simulink model "Pole_Placement_Digital_a"  (Simulink 9.0)
settings: Solver=VariableStepAuto  StartTime=0.0  StopTime=60  RelTol=1e-3
values from neighbouring files (symbols this model uses):
  C_D2 = c2d(C2_aug, T, 'tustin')    [Lab3_Pole_Placement_Integrator.m]
  K1 = 0.66538    [Lab3_Pole_Placement_Integrator.m]
  K2 = 0.062    [Lab3_Pole_Placement_Integrator.m]
  K3 = 4.78    [Lab3_Pole_Placement_Integrator.m]
  Kp = 15    [Lab3_Pole_Placement_Integrator.m]
  Kp_c2 = 2 / DC_gain    [Lab3_Pole_Placement_Integrator.m]
  p = 10.5    [Lab3_Pole_Placement_Integrator.m]
  T = 0.005    [Lab3_Pole_Placement_Integrator.m]
  tau = 0.030541    [Lab3_Pole_Placement_Integrator.m]
  z = 10    [Lab3_Pole_Placement_Integrator.m]
settings Model: Creator=joe  LastModifiedBy=joe
settings DataIOCC: SaveFormat=Dataset
settings DebuggingCC: UnderspecifiedInitializationDetection=Simplified  MergeDetectMultiDrivingBlocksExec=error  SFUnexpectedBacktrackingDiag=error  SFNoUnconditionalDefaultTransitionDiag=error
settings HardwareCC: ProdBitPerPointer=64  ProdBitPerSizeT=64  ProdBitPerPtrDiffT=64  ProdLargestAtomicFloat=Float  ProdIntDivRoundTo=Zero  ProdEndianess=LittleEndian  ProdWordSize=64  ProdHWDeviceType=Intel->x86-64 (Windows64)
settings ModelReferenceCC: PropagateSignalLabelsOutOfModel=on
settings GRTTargetCC: TargetLangStandard=C99 (ISO)
settings ConfigComp: CovMetricSettings=dwe  CovHtmlReporting=off  CovSaveCumulativeToWorkspaceVar=off  CovSaveSingleToWorkspaceVar=off  CovExternalEMLEnable=on

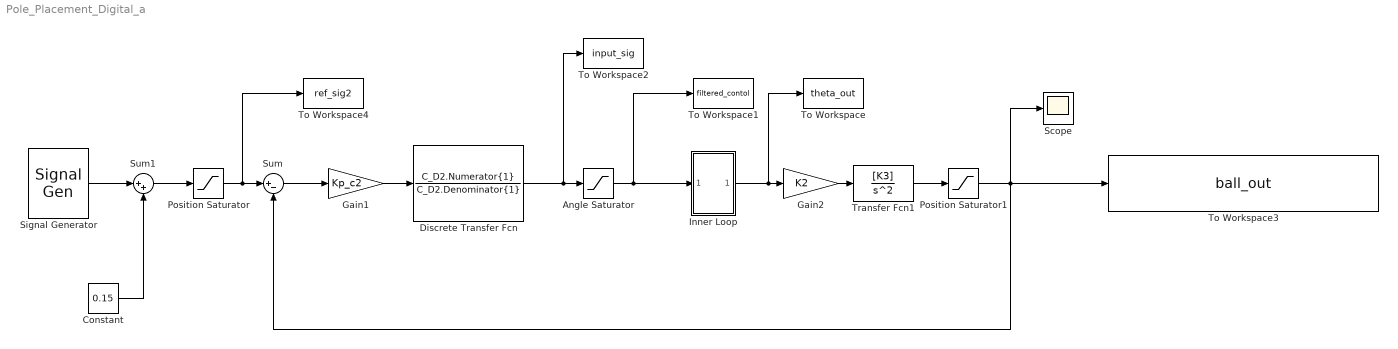
== system Pole_Placement_Digital_a ==
  Angle Saturator : Saturate  UpperLimit=0.785  LowerLimit=-0.785
  Constant : Constant  Value=0.15
  Discrete Transfer Fcn : DiscreteTransferFcn  Numerator=C_D2.Numerator{1}  Denominator=C_D2.Denominator{1}  SampleTime=T
  Gain1 : Gain  Gain=Kp_c2
  Gain2 : Gain  Gain=K2
  Inner Loop : Subsystem
  Position Saturator : Saturate  UpperLimit=0.417  LowerLimit=0
  Position Saturator1 : Saturate  UpperLimit=0.417  LowerLimit=0
  Scope : Scope
  Signal Generator : SignalGenerator  WaveForm=square  Amplitude=0.03  Frequency=0.05
  Sum : Sum  Inputs=|+-
  Sum1 : Sum  Inputs=|++
  To Workspace : ToWorkspace  VariableName=theta_out  SaveFormat=Timeseries  SampleTime=-1
  To Workspace1 : ToWorkspace  VariableName=filtered_contol  SaveFormat=Timeseries  SampleTime=-1
  To Workspace2 : ToWorkspace  VariableName=input_sig  SaveFormat=Timeseries  SampleTime=-1
  To Workspace3 : ToWorkspace  VariableName=ball_out  SaveFormat=Timeseries  SampleTime=-1
  To Workspace4 : ToWorkspace  VariableName=ref_sig2  SaveFormat=Timeseries  SampleTime=-1
  Transfer Fcn1 : TransferFcn  Numerator=[K3]  Denominator=[1 0 0]
  wires:
  Discrete Transfer Fcn/1 -> To Workspace2/1, Angle Saturator/1
  Angle Saturator/1 -> To Workspace1/1, Inner Loop/1(In1)
  Gain1/1 -> Discrete Transfer Fcn/1
  Sum/1 -> Gain1/1
  Position Saturator/1 -> To Workspace4/1, Sum/1
  Gain2/1 -> Transfer Fcn1/1
  Inner Loop/1(Out1) -> To Workspace/1, Gain2/1
  Transfer Fcn1/1 -> Position Saturator1/1
  Signal Generator/1 -> Sum1/1
  Sum1/1 -> Position Saturator/1
  Constant/1 -> Sum1/2
  Position Saturator1/1 -> Sum/2, To Workspace3/1, Scope/1

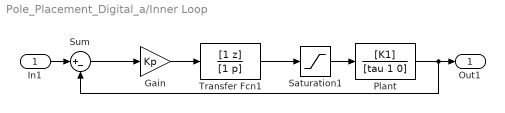
== system Pole_Placement_Digital_a/Inner Loop ==
  In1 : Inport
  Gain : Gain  Gain=Kp
  Plant : TransferFcn  Numerator=[K1]  Denominator=[tau 1 0]
  Saturation1 : Saturate  UpperLimit=6  LowerLimit=-6
  Sum : Sum  Inputs=|+-
  Transfer Fcn1 : TransferFcn  Numerator=[1 z]  Denominator=[1 p]
  Out1 : Outport
  wires:
  In1/1 -> Sum/1
  Plant/1 -> Sum/2, Out1/1
  Gain/1 -> Transfer Fcn1/1
  Transfer Fcn1/1 -> Saturation1/1
  Sum/1 -> Gain/1
  Saturation1/1 -> Plant/1
